simulink model "RL_NL_simulation"  (R2024b)
settings: Solver=VariableStepAuto  StartTime=0.0  StopTime=10.0  RelTol=1e-3
values from neighbouring files (symbols this model uses):
  g = 9.81    [PI_requirement.m]    (also in RL_model.m)
  i_e = sqrt((m*g/km) * (x_e + 2*r -l)^2)    [RL_model.m]
  Kg = 3    [PI_requirement.m]    (also in RL_model.m)
  Ki_i = Kp_i/Ti    [RL_model.m]
  km = 6.5308e-5    (= 6.5308e-05)    [PI_requirement.m]    (also in RL_model.m)
  Kp_i = sqrt(R^2 + (wc*L)^2) / ( Kg * sqrt(1 + 1/(wc^2 * Ti^2)) )    [RL_model.m]
  l = 0.0394    [PI_requirement.m]    (also in RL_model.m)
  L = 412.5e-3    (= 0.4125)    [PI_requirement.m]    (also in RL_model.m)
  m = 0.068    [PI_requirement.m]    (also in RL_model.m)
  r = 1.27e-2    (= 0.0127)    [PI_requirement.m]    (also in RL_model.m)
  R = (Rc + Rs)* Rcal    (= 9.35)    [PI_requirement.m]    (also in RL_model.m)
  x_e = l/2 - r    (= 0.007)    [RL_model.m]
undefined symbols (not defined in the file or in its folder): G_i_den, G_i_num
libraries: slpidlib x1
settings Model: Creator=edoardo  LastModifiedBy=edoardo

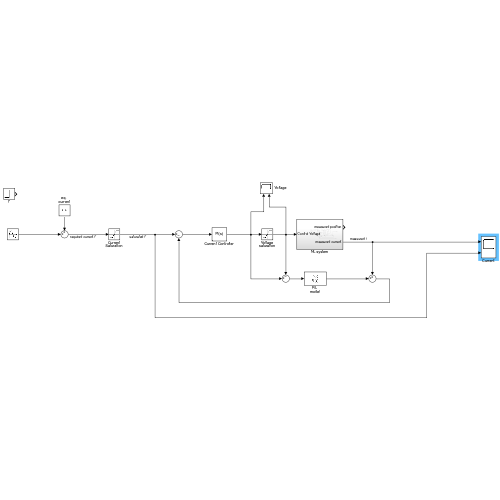
[thumbnail: Simulink's stored preview of the top-level diagram]
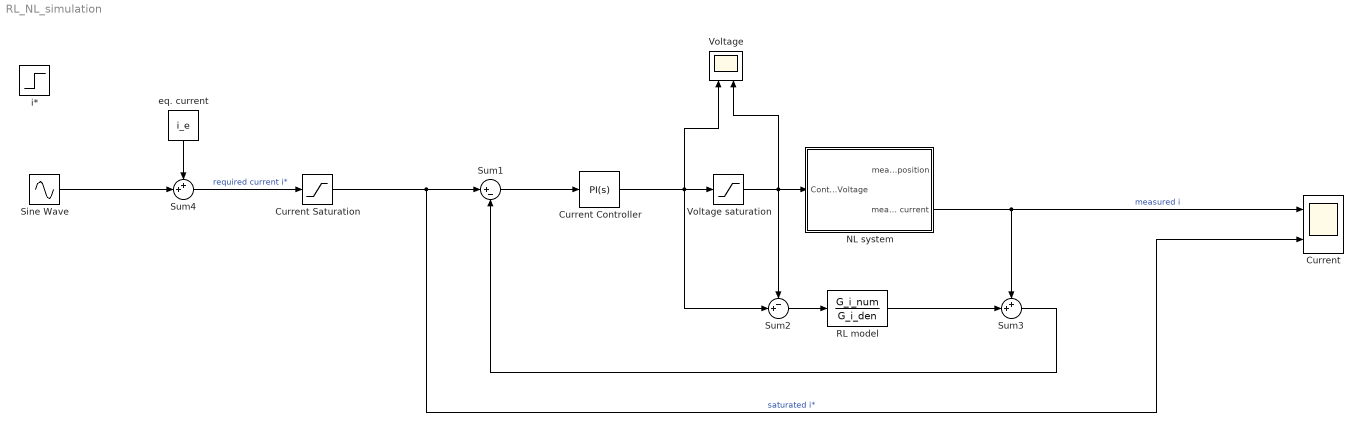
== system RL_NL_simulation ==
  Current : Scope  NumInputPorts=2
  Current Saturation : Saturate  UpperLimit=3  LowerLimit=-3
  Current Controller : slpidlib/PID Controller  Controller=PI  Form=Parallel  TimeDomain=Continuous-time  UseExternalTs=off  SampleTime=-1  IntegratorMethod=Forward Euler  FilterMethod=Forward Euler  ControllerParametersSource=internal  P=Kp_i  I=Ki_i  UseKiTs=off  D=0  UseExternalDerivativeSource=off  N=100  UseFilter=on  TunerSelectOption=Transfer Function Based (PID Tuner App)  InitialConditionSource=internal  InitialConditionForIntegrator=0  InitialConditionForFilter=0  DifferentiatorICPrevScaledInput=0  ExternalReset=none  TrackingMode=off  Kt=1  LimitOutput=off  SatLimitsSource=internal  UpperSaturationLimit=inf  LowerSaturationLimit=-inf  LinearizeAsGain=on  AntiWindupMode=none  Kb=1  LimitIntegrator=off  UpperIntegratorSaturationLimit=inf  LowerIntegratorSaturationLimit=-inf  POutMin=[]  POutMax=[]  IOutMin=[]  IOutMax=[]  DOutMin=[]  DOutMax=[]  NOutMin=[]  NOutMax=[]  SumOutMin=[]  SumOutMax=[]  SaturationOutMin=[]  SaturationOutMax=[]  PParamMin=[]  PParamMax=[]  IParamMin=[]  IParamMax=[]  DParamMin=[]  DParamMax=[]  NParamMin=[]  NParamMax=[]  KbParamMin=[]  KbParamMax=[]  KtParamMin=[]  KtParamMax=[]  KbOutMin=[]  KbOutMax=[]  KtOutMin=[]  KtOutMax=[]  IntegratorOutMin=[]  IntegratorOutMax=[]  FilterOutMin=[]  FilterOutMax=[]  SumI1OutMin=[]  SumI1OutMax=[]  SumI2OutMin=[]  SumI2OutMax=[]  SumI3OutMin=[]  SumI3OutMax=[]  SumI4OutMin=[]  SumI4OutMax=[]  SumDOutMin=[]  SumDOutMax=[]  DifferentiatorOutMin=[]  DifferentiatorOutMax=[]  FilterDiffOutCoefMin=[]  FilterDiffOutCoefMax=[]  ReciprocalOutMin=[]  ReciprocalOutMax=[]  SumDenOutMin=[]  SumDenOutMax=[]  SumNumOutMin=[]  SumNumOutMax=[]  DivideOutMin=[]  DivideOutMax=[]  UdiffTsProdOutMin=[]  UdiffTsProdOutMax=[]  NTsProdOutMin=[]  NTsProdOutMax=[]  UintegralTsProdOutMin=[]  UintegralTsProdOutMax=[]  UngainTsProdOutMin=[]  UngainTsProdOutMax=[]  ClampingZeroOutDataTypeStr=Inherit: Inherit via back propagation  ClampingZeroOutMin=[]  ClampingZeroOutMax=[]  FilterDenConstantOutDataTypeStr=Inherit: Inherit via back propagation  FilterDenConstantOutMin=[]  FilterDenConstantOutMax=[]  PCopyOutDataTypeStr=Inherit: Inherit via back propagation  PCopyOutMin=[]  PCopyOutMax=[]  NCopyOutDataTypeStr=Inherit: Inherit via back propagation  NCopyOutMin=[]  NCopyOutMax=[]  IntegratorContinuousStateAttributes=''  IntegratorStateMustResolveToSignalObject=off  IntegratorRTWStateStorageClass=Auto  FilterContinuousStateAttributes=''  FilterStateMustResolveToSignalObject=off  FilterRTWStateStorageClass=Auto  ParallelPVariant=InternalParameters  IdealPVariant=Disabled  IVariant=InternalParameters  DVariant=Disabled  IntegratorVariant=Continuous  SatVariant=Disabled  AWVariant=Passthrough  PCopyVariant=Disabled  TRVariant=Disabled  FdbkBlocksVariant=Forward  IdealPFdbkVariant=Disabled  SatFdbkVariant=Disabled  DerivativeFilterVariant=Disabled  NVariant=Disabled  NCopyVariant=Disabled_SignalSpec  FilterICVariant=Disabled  IntegratorICVariant=InternalICs  ExternalResetVariant=Disabled  TRSumVariant=Passthrough  SumFdbkVariant=Disabled  SumVariant=Sum_PI  TsampFilterVariant=InternalTs  TsampNgainVariant=Passthrough  TsampIntegralVariant=Disabled_SignalSpec  ExternalSaturationOutDataTypeStr=Inherit: Same as second input  DerivativeSourceVariant=Disabled  PreIntVariant=InternalPreInt
  NL system : Subsystem
  RL model : TransferFcn  Numerator=G_i_num  Denominator=G_i_den
  Sine Wave : Sin  Amplitude=0.7  Frequency=20  SampleTime=0
  Sum1 : Sum  Inputs=|+-
  Sum2 : Sum  Inputs=-+|
  Sum3 : Sum  Inputs=++|
  Sum4 : Sum  Inputs=++|
  Voltage : Scope  NumInputPorts=2
  Voltage saturation : Saturate  UpperLimit=8  LowerLimit=-8
  eq. current : Constant  Value=i_e
  i* : Step  After=0  SampleTime=0
  wires:
  Current Controller/1 -> Voltage/1, Sum2/2, Voltage saturation/1
  RL model/1 -> Sum3/2
  Sum3/1 -> Sum1/2
  Sum2/1 -> RL model/1
  Voltage saturation/1 -> NL system/1(Control Voltage), Voltage/2, Sum2/1
  Sum1/1 -> Current Controller/1
  Current Saturation/1 -> Sum1/1, Current/2  "saturated i*"
  eq. current/1 -> Sum4/1
  NL system/2(measured current) -> Sum3/1, Current/1  "measured i"
  Sum4/1 -> Current Saturation/1  "required current i*"
  Sine Wave/1 -> Sum4/2

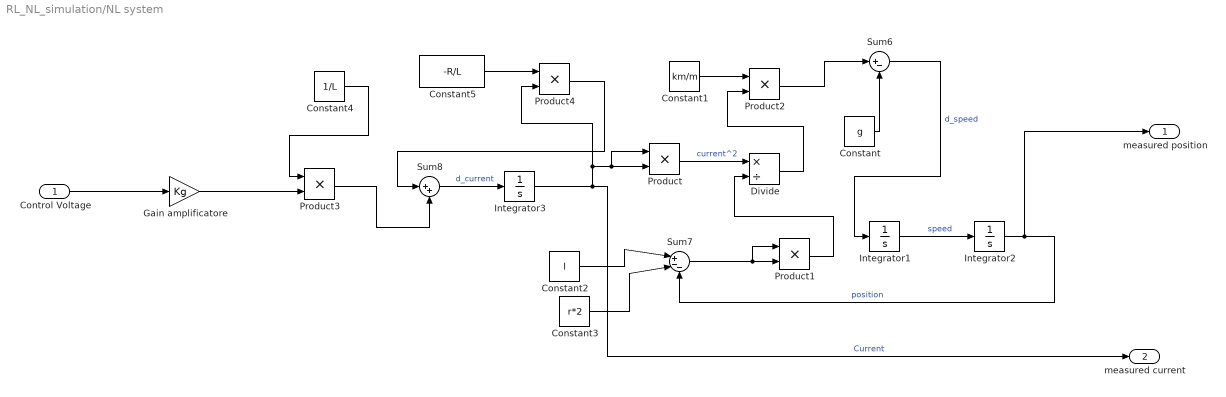
== system RL_NL_simulation/NL system ==
  Control Voltage : Inport
  Constant : Constant  Value=g
  Constant1 : Constant  Value=km/m
  Constant2 : Constant  Value=l
  Constant3 : Constant  Value=r*2
  Constant4 : Constant  Value=1/L
  Constant5 : Constant  Value=-R/L
  Divide : Product  Inputs=*/
  Gain amplificatore : Gain  Gain=Kg
  Integrator1 : Integrator
  Integrator2 : Integrator  InitialCondition=x_e  LimitOutput=on  LowerSaturationLimit=0
  Integrator3 : Integrator
  Product{,1..4} (5 alike) : Product
  Sum6 : Sum  Inputs=|+-
  Sum7 : Sum  Inputs=|+--
  Sum8 : Sum  Inputs=|++
  measured position : Outport
  measured current : Outport  Port=2
  wires:
  Divide/1 -> Product2/2
  Constant3/1 -> Sum7/2
  Constant/1 -> Sum6/2
  Sum6/1 -> Integrator1/1  "d_speed"
  Constant1/1 -> Product2/1
  Product/1 -> Divide/1  "current^2"
  Control Voltage/1 -> Gain amplificatore/1
  Product4/1 -> Sum8/1
  Product1/1 -> Divide/2
  Sum7/1 -> Product1/2, Product1/1
  Product3/1 -> Sum8/2
  Integrator1/1 -> Integrator2/1  "speed"
  Constant4/1 -> Product3/1
  Product2/1 -> Sum6/1
  Constant5/1 -> Product4/1
  Sum8/1 -> Integrator3/1  "d_current"
  Integrator2/1 -> measured position/1, Sum7/3  "position"
  Constant2/1 -> Sum7/1
  Integrator3/1 -> measured current/1, Product4/2, Product/2, Product/1  "Current"
  Gain amplificatore/1 -> Product3/2
